simulink model "Control_BA"  (R2023b)
settings: Solver=FixedStepAuto  StartTime=0.0  StopTime=12.0  RelTol=1e-3  EnableMultiTasking=on
settings Model: ExtModeTrigDuration=2  Creator=Enrique  LastModifiedBy=Enrique
settings OptimizationCC: EnhancedBackFolding=on  PassReuseOutputArgsAs=Individual arguments  ZeroExternalMemoryAtStartup=off  ZeroInternalMemoryAtStartup=off  MaxStackSize=64  OptimizeBlockOrder=speed  DifferentSizesBufferReuse=on  OptimizationCustomize=off  EfficientTunableParamExpr=on
settings DebuggingCC: ParameterTunabilityLossMsg=error
settings HardwareCC: ProdBitPerInt=16  ProdBitPerPointer=16  ProdBitPerSizeT=16  ProdBitPerPtrDiffT=16  ProdLargestAtomicFloat=None  ProdWordSize=8  ProdHWDeviceType=Atmel->AVR  UseEmbeddedCoderFeatures=off  UseSimulinkCoderFeatures=off
settings SFSimCC: MATLABDynamicMemAlloc=off
settings RTWCC: Description=Embedded Coder  SystemTargetFile=ert.tlc  HardwareBoard=Arduino Mega 2560  TemplateMakefile=ert_default_tmf  Toolchain=Arduino AVR  BuildConfiguration=Faster Runs
settings CodeAppCC: ForceParamTrailComments=on  IgnoreCustomStorageClasses=off  OperatorAnnotations=on  SimulinkDataObjDesc=on  SFDataObjDesc=on  InsertBlockDesc=on
settings ERTTargetCC: SupportContinuousTime=on  SupportNonInlinedSFcns=on  SupportVariableSizeSignals=on  ExtModeTransport=3  ExtModeStaticAlloc=on  ExtModeAutomaticAllocSize=off  ExtModeStaticAllocSize=2048  ExtModeMexFile=ext_xcp  ExtModeIntrfLevel=Level2 - Open

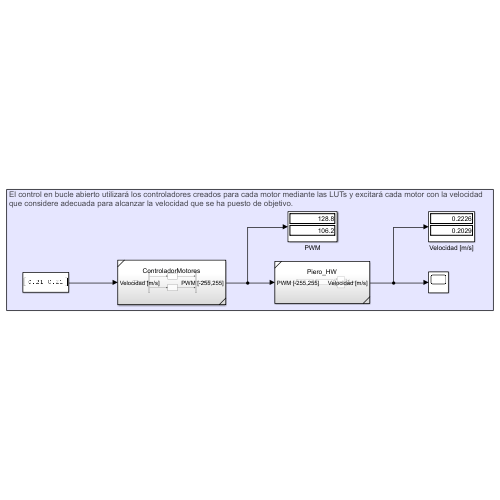
[thumbnail: Simulink's stored preview of the top-level diagram]
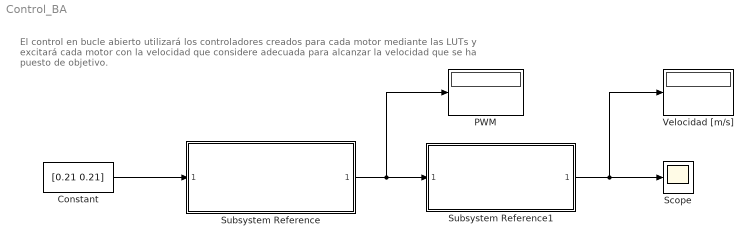
== system Control_BA ==
  note: El control en bucle abierto utilizará los controladores creados para cada motor mediante las LUTs y excitará cada motor con la velocidad
      | que considere adecuada para alcanzar la velocidad que se ha puesto de objetivo.
  Constant : Constant  Value=[0.21 0.21]
  PWM : Display
  Scope : Scope
  Subsystem Reference : Subsystem  ReferencedSubsystem=ControladorMotores
  Subsystem Reference1 : Subsystem  ReferencedSubsystem=Piero_HW
  Velocidad [m/s] : Display
  wires:
  Subsystem Reference/1 -> PWM/1, Subsystem Reference1/1
  Subsystem Reference1/1 -> Velocidad [m/s]/1, Scope/1
  Constant/1 -> Subsystem Reference/1
